simulink model "pendulum_model_1000mAh"  (R2017a)
settings: Solver=FixedStepAuto  StartTime=0.0  StopTime=10  FixedStep=0.01  RelTol=1e-3
values from neighbouring files (symbols this model uses):
  c = 1.83e-04    (= 0.000183)    [Swing_Test_Graph_1000mAh.m]
  g = 9.81    [Swing_Test_Graph_1000mAh.m]    (also in leastSquares.m; odeSolve.m)
  I = 4.4e-03    (= 0.0044)    [Swing_Test_Graph_1000mAh.m]
  len = 0.093    [Swing_Test_Graph_1000mAh.m]
  M = 0.330    (= 0.33)    [Swing_Test_Graph_1000mAh.m]    (also in leastSquares.m; odeSolve.m = 0.352)
  theta0 = 0.83    [Swing_Test_Graph_1000mAh.m]
settings Model: Creator=Patrick  LastModifiedBy=Patrick
settings DataIOCC: TimeSaveName=tsim

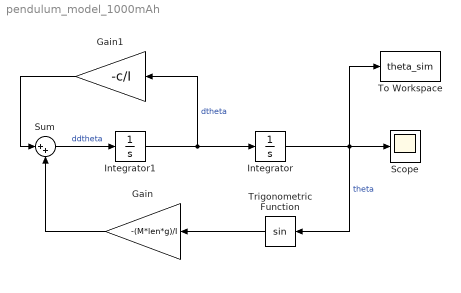
== system pendulum_model_1000mAh ==
  Gain : Gain  Gain=-(M*len*g)/I
  Gain1 : Gain  Gain=-c/I
  Integrator : Integrator  InitialCondition=theta0
  Integrator1 : Integrator
  Scope : Scope
  Sum : Sum  Inputs=|++
  To Workspace : ToWorkspace  VariableName=theta_sim  SampleTime=-1
  Trigonometric Function : Trigonometry
  wires:
  Integrator/1 -> To Workspace/1, Scope/1, Trigonometric Function/1  "theta"
  Integrator1/1 -> Integrator/1, Gain1/1  "dtheta"
  Trigonometric Function/1 -> Gain/1
  Sum/1 -> Integrator1/1  "ddtheta"
  Gain1/1 -> Sum/1
  Gain/1 -> Sum/2
